simulink model "Stop_and_Wait"  (R2024b)
settings: Solver=FixedStepDiscrete  StartTime=0.0  StopTime=10.0  FixedStep=0.1  RelTol=1e-3  EnableMultiTasking=on
model workspace (MAT data in the model file):
  TxTree : serdes.internal.ibisami.ami.SerDesTree (value not decoded)
  input = Simulink.Bus
  input.Alignment = -1
  input.PreserveElementDimensions = 0
  input.Elements_internal = Simulink.BusElement
  input.Elements_internal.DimensionsMode = 'Fixed'
  input.Elements_internal.SamplingMode = 'Sample based'
  input.Elements_internal.SampleTime = -1
  input.Elements_internal.Name = 'in_data'
  input.Elements_internal.DataType_internal = 'uint8'
  input.Elements_internal.Complexity = 'real'
  input.Elements_internal.Dimensions = 1
  input.DataScope = 'Auto'
  output = Simulink.Bus
  output.Alignment = -1
  output.PreserveElementDimensions = 0
  output.Elements_internal = Simulink.BusElement
  output.Elements_internal.DimensionsMode = 'Fixed'
  output.Elements_internal.SamplingMode = 'Sample based'
  output.Elements_internal.SampleTime = -1
  output.Elements_internal.Name = 'out_data'
  output.Elements_internal.DataType_internal = 'uint8'
  output.Elements_internal.Complexity = 'real'
  output.Elements_internal.Dimensions = 1
  output.DataScope = 'Auto'
libraries: instrumentlib x4, dspbuff3 x1, simulink x1
settings Model: Creator=Amin  LastModifiedBy=Amin
settings SolverCC: PositivePriorityOrder=on
settings OptimizationCC: DefaultParameterBehavior=Inlined  EnhancedBackFolding=on  PassReuseOutputArgsAs=Individual arguments  ZeroExternalMemoryAtStartup=off  ZeroInternalMemoryAtStartup=off  MaxStackSize=64  OptimizeBlockOrder=speed  DifferentSizesBufferReuse=on  OptimizationCustomize=off  EfficientTunableParamExpr=on
settings DebuggingCC: ParameterTunabilityLossMsg=error
settings HardwareCC: ProdLongLongMode=on
settings ModelReferenceCC: ModelReferenceNumInstancesAllowed=Single
settings SFSimCC: LegacyBehaviorForPersistentVarInContinuousTime=on
settings RTWCC: Description=Embedded Coder  SystemTargetFile=ert.tlc  GenCodeOnly=on  PackageGeneratedCodeAndArtifacts=on  TemplateMakefile=ert_default_tmf  TargetLang=C++
settings CodeAppCC: ForceParamTrailComments=on  IgnoreCustomStorageClasses=off  OperatorAnnotations=on  SimulinkDataObjDesc=on  SFDataObjDesc=on  InsertBlockDesc=on
settings ERTTargetCC: CodeInterfacePackaging=C++ class  RootIOFormat=Structure reference  RTWCAPIRootIO=on  ERTCustomFileTemplate=example_file_process.tlc

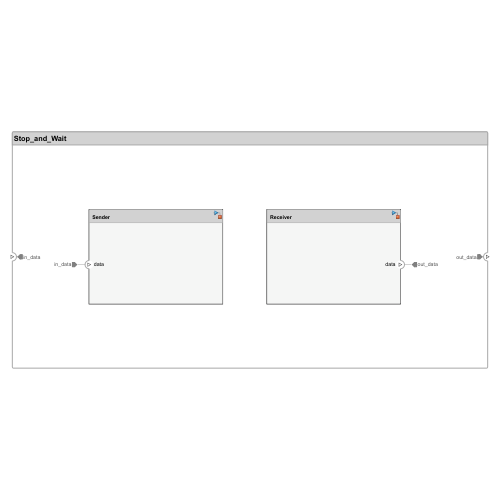
[thumbnail: Simulink's stored preview of the top-level diagram]
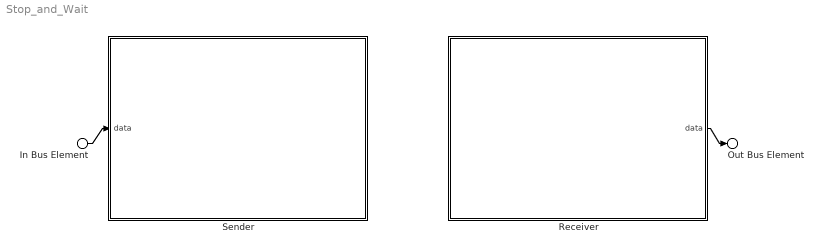
== system Stop_and_Wait ==
  In Bus Element : Inport  PortName=in_data
  Receiver : Subsystem
      settings: PortSchema="{\"entries\":[{\"content\":{\"headerSize\":26,\"margin\":15,\"minimumSpacing\":25,\"sides\":[{\"content\":{},\"type\":\"ConnectorPlacement.EquallySpacedRectSide\",\"uuid\":\"0072a2cb-bb3d-48a2-9d64-8e46ce8a1590\"},{\"content\":{\"connectorIds\":[\"Out1\"],\"side\":\"RIGHT\"},\"type\":\"ConnectorPlacement.EquallySpacedRectSide\",\"uuid\":\"e1929af3-b524-4cb4-8bf7-a19049f030de\"},{\"content\":{\"side\":\"TOP\"},\"type\":\"ConnectorPlacement.EquallySpacedRectSide\",\"uuid\":\"578aca91-09af-4b8b-8516-407c0ce534ed\"}]},\"type\":\"ConnectorPlacement.EquallySpacedConnector\",\"uuid\":\"ac7dd36b-d2bb-4d4d-8d57-dee4a1353f16\"}],\"packageUris\":[\"http://schema.mathworks.com/mf0/Connector/R2020b\"],\"version\":\"1.0\"}"
  Sender : Subsystem
      settings: PortSchema="{\"entries\":[{\"content\":{\"headerSize\":26,\"margin\":15,\"minimumSpacing\":25,\"sides\":[{\"content\":{\"connectorIds\":[\"In1\"]},\"type\":\"ConnectorPlacement.EquallySpacedRectSide\",\"uuid\":\"0072a2cb-bb3d-48a2-9d64-8e46ce8a1590\"},{\"content\":{\"side\":\"RIGHT\"},\"type\":\"ConnectorPlacement.EquallySpacedRectSide\",\"uuid\":\"e1929af3-b524-4cb4-8bf7-a19049f030de\"},{\"content\":{\"side\":\"TOP\"},\"type\":\"ConnectorPlacement.EquallySpacedRectSide\",\"uuid\":\"578aca91-09af-4b8b-8516-407c0ce534ed\"}]},\"type\":\"ConnectorPlacement.EquallySpacedConnector\",\"uuid\":\"ac7dd36b-d2bb-4d4d-8d57-dee4a1353f16\"}],\"packageUris\":[\"http://schema.mathworks.com/mf0/Connector/R2020b\"],\"version\":\"1.0\"}"
  Out Bus Element : Outport  PortName=out_data
  wires:
  In Bus Element/1 -> Sender/1(data)
  Receiver/1(data) -> Out Bus Element/1

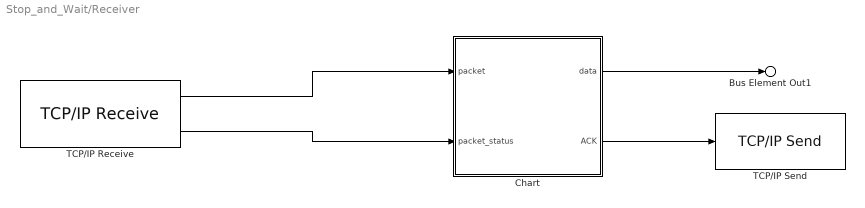
== system Stop_and_Wait/Receiver ==
  Chart : Stateflow chart  TreatAsAtomicUnit=on
  TCP/IP Receive : instrumentlib/TCP//IP Receive  Host=localhost  Port=54321  DataSize=[1, 1]  DataType=uint16  ASCIIFormatting=%f  Terminator=LF  CustomTerminator=10  ByteOrder=big-endian  EnableBlockingMode=off  Timeout=4  SampleTime=0.1  SimulateUsing=Interpreted execution
  TCP/IP Send : instrumentlib/TCP//IP Send  Host=localhost  Port=12345  ByteOrder=big-endian  EnableBlockingMode=off  Timeout=10  TransferDelay=off  SimulateUsing=Interpreted execution
  Bus Element Out1 : Outport  PortName=data  Element=out_data
  wires:
  Chart/2(ACK) -> TCP/IP Send/1
  Chart/1(data) -> Bus Element Out1/1
  TCP/IP Receive/1 -> Chart/1(packet)
  TCP/IP Receive/2 -> Chart/2(packet_status)

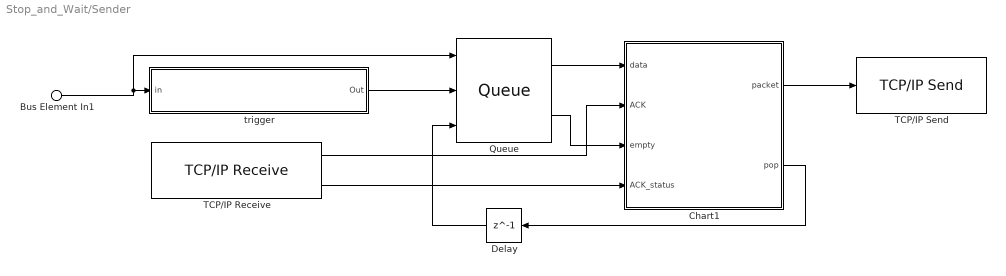
== system Stop_and_Wait/Sender ==
  Bus Element In1 : Inport  PortName=data  Element=in_data
  Chart1 : Stateflow chart  TreatAsAtomicUnit=on
  Delay : Delay  DelayLength=1
  Queue : dspbuff3/Queue  depth=256  trigger=Either edge  overflow=Warning  pes=Warning  eso=on  fso=off  nso=off  clr=off  clrOutport=off  adf=on
  TCP/IP Receive : instrumentlib/TCP//IP Receive  Host=localhost  Port=12345  DataSize=[1, 1]  DataType=uint8  ASCIIFormatting=%f  Terminator=LF  CustomTerminator=10  ByteOrder=big-endian  EnableBlockingMode=off  Timeout=4  SampleTime=0.1  SimulateUsing=Interpreted execution
  TCP/IP Send : instrumentlib/TCP//IP Send  Host=localhost  Port=54321  ByteOrder=big-endian  EnableBlockingMode=off  Timeout=4  TransferDelay=off  SimulateUsing=Interpreted execution
  trigger : Subsystem
  wires:
  TCP/IP Receive/1 -> Chart1/2(ACK)
  Chart1/1(packet) -> TCP/IP Send/1
  Queue/1 -> Chart1/1(data)
  Queue/2 -> Chart1/3(empty)
  Delay/1 -> Queue/3
  Chart1/2(pop) -> Delay/1
  trigger/1(Out) -> Queue/2
  TCP/IP Receive/2 -> Chart1/4(ACK_status)
  Bus Element In1/1 -> Queue/1, trigger/1(in)

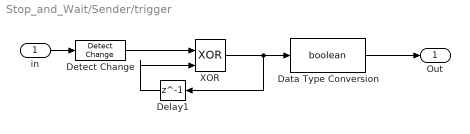
== system Stop_and_Wait/Sender/trigger ==
  in : Inport
  Data Type Conversion : DataTypeConversion  OutDataTypeStr=boolean  SaturateOnIntegerOverflow=off  RndMeth=Floor
  Delay1 : Delay  DelayLength=1
  Detect Change : simulink/Logic and Bit Operations/Detect Change  vinit=0  OutDataTypeStr=uint8
  XOR : Logic  Operator=XOR  IconShape=distinctive  AllPortsSameDT=off  OutDataTypeStr=boolean
  Out : Outport
  wires:
  XOR/1 -> Delay1/1, Data Type Conversion/1
  Delay1/1 -> XOR/2
  Detect Change/1 -> XOR/1
  Data Type Conversion/1 -> Out/1
  in/1 -> Detect Change/1

== stateflow chart Stop_and_Wait/Sender/Chart1 ==
  settings: stateMachineType=MEALY_MACHINE  executeAtInitialization=1
  state Dequeue
  state Send_packet
  state Wait_for_ack
  (default) -> Send_packet
  Dequeue -> Wait_for_ack : {packet = uint16(calculation(data, tag))}
  Send_packet -> Dequeue : [~empty]{send(pop)}
  Wait_for_ack -> Send_packet [order 2] : [ACK_status == 1 && checkACK(ACK, c_ACK)]{c_ACK = c_ACK + 1; tag = 1-tag;}
  Wait_for_ack -> Wait_for_ack [order 1] : [after(TIMEOUT, sec)]{packet = uint16(calculation(data, tag));}
  data: f function_output; ack function_input; check function_input; value function_input; t function_input; header function_output; polynomial function_input; input function_input uint8; output function_output uint16; c_tag function_input; value function_input; header function_output; polynomial function_input; TIMEOUT constant double =4; packet output uint16; data input uint8; ACK input uint8; c_ACK local uint8 =1; empty input boolean; ACK_status input; tag local single =1
  events: pop output EITHER_EDGE_EVENT
  function f = checkACK(ack, check):
    | function f = checkACK(ack, check)
    | 
    |     header = uint8(bitshift(ack, -4));
    |     ack_value = uint8(bitand(ack, 0x0F));
    |     if ack_crc(ack_value, 19) == header && ack_value == check
    |         f = true;
    |     else
    |         f = false;
    |     end
    |     
    | end
  function header = crc4(value, t, polynomial):
    | function header = crc4(value, t, polynomial)
    |         
    |     % Initialize the CRC register to 0
    |     crc = uint16(0);
    |     input = bitor(uint16(value), bitshift(uint16(t), 8));
    |         
    |     % Loop over each bit in the input byte (MSB first)
    |     for i = 8:-1:-4
    |         % XOR the MSB of the input with the MSB of the CRC register
    |         crc = bitxor(crc, bitand(bitshift(input, -i), 1));  % Shift input and XOR
    |             
    |         % If the MSB of the CRC is 1, perform the polynomial division (XOR)
    |         if bitget(crc, 5)  % Check if MSB (bit 5) of 8-bit crc is set
    |            crc = bitxor(crc, polynomial);  % Perform division by XOR with polynomial
    |         end
    |             
    |         if i ~= -4
    |             % Shift CRC register left by 1 bit
    |             crc = bitshift(crc, 1);
    |         end
    |     end
    |         
    |     
    |     % Final CRC value is the remainder in the lowest 4 bits
    |     header = uint8(bitand(crc, 15));  % Mask to get the lower 4 bits as the CRC result
    | end
  function output = calculation(input, c_tag):
    | function output = calculation(input, c_tag)
    |     
    |     
    |     output = bitor(bitor(uint16(input), bitshift(uint16(c_tag), 8)), bitshift(uint16(crc4(input, c_tag, 19)), 9));
    | 
    | end
  function header = ack_crc(value, polynomial):
    | function header = ack_crc(value, polynomial)
    |         
    |     % Initialize the CRC register to 0
    |     crc = uint8(0);
    |         
    |     % Loop over each bit in the input byte (MSB first)
    |     for i = 7:-1:-4
    |         % XOR the MSB of the input with the MSB of the CRC register
    |         crc = bitxor(crc, bitand(bitshift(value, -i), 1));  % Shift input and XOR
    |             
    |         % If the MSB of the CRC is 1, perform the polynomial division (XOR)
    |         if bitget(crc, 5)  % Check if MSB (bit 5) of 8-bit crc is set
    |            crc = bitxor(crc, polynomial);  % Perform division by XOR with polynomial
    |         end
    |             
    |         if i ~= -4
    |             % Shift CRC register left by 1 bit
    |             crc = bitshift(crc, 1);
    |         end
    |     end
    |         
    |     
    |     % Final CRC value is the remainder in the lowest 4 bits
    |     header = bitand(crc, 15);  % Mask to get the lower 4 bits as the CRC result
    | end

== stateflow chart Stop_and_Wait/Receiver/Chart ==
  settings: executeAtInitialization=1
  state state
  (default) -> state
  state -> state : [packet_status == 1 && check_packet(packet, tag)]{[data, ACK, c_ack] = send_data_ack(packet, c_ack); tag = 1-tag}
  data: f function_output; p function_input; t function_input; value function_input; crc_tag function_input; header function_output; polynomial function_input; p function_input; d function_output; a function_output; c function_input; nc function_output; value function_input; header function_output; polynomial function_input; data output uint8 =0; packet input uint16; ACK output uint8 =0; c_ack local uint8 =0; packet_status input boolean; tag local single =1
  function f = check_packet(p, t):
    | function f = check_packet(p, t)
    | 
    |     header = uint8(bitshift(p, -9));
    |     raw_data = uint8(bitand(p, 0x00FF));
    |     checktag = bitget(p, 9);
    |     if crc4(raw_data, tag, 19) == header && checktag == t
    |         f = true;
    |     else
    |         f = false;
    |     end
    |     
    | end
  function header = crc4(value, crc_tag, polynomial):
    | function header = crc4(value, crc_tag, polynomial)
    |         
    |     % Initialize the CRC register to 0
    |     crc = uint16(0);
    |     input = bitor(uint16(value), bitshift(uint16(crc_tag), 8));
    |         
    |     % Loop over each bit in the input byte (MSB first)
    |     for i = 8:-1:-4
    |         % XOR the MSB of the input with the MSB of the CRC register
    |         crc = bitxor(crc, bitand(bitshift(input, -i), 1));  % Shift input and XOR
    |             
    |         % If the MSB of the CRC is 1, perform the polynomial division (XOR)
    |         if bitget(crc, 5)  % Check if MSB (bit 5) of 8-bit crc is set
    |            crc = bitxor(crc, polynomial);  % Perform division by XOR with polynomial
    |         end
    |             
    |         if i ~= -4
    |             % Shift CRC register left by 1 bit
    |             crc = bitshift(crc, 1);
    |         end
    |     end
    |         
    |     
    |     % Final CRC value is the remainder in the lowest 4 bits
    |     header = uint8(bitand(crc, 15));  % Mask to get the lower 4 bits as the CRC result
    | end
  function [d, a, nc]= send_data_ack(p, c):
    | function [d, a, nc]= send_data_ack(p, c)
    | 
    |     d = uint8(bitand(p, 0x0011));
    | 
    |     if c == 16
    |         nc = uint8(0);
    |     else
    |         nc = uint8(c+1);
    |     end
    | 
    |     a = bitor(uint8(c+1), bitshift(uint8(ack_crc(uint8(c+1), 19)), 4));
    | 
    | end
  function header = ack_crc(value, polynomial):
    | function header = ack_crc(value, polynomial)
    |         
    |     % Initialize the CRC register to 0
    |     crc = uint8(0);
    |         
    |     % Loop over each bit in the input byte (MSB first)
    |     for i = 7:-1:-4
    |         % XOR the MSB of the input with the MSB of the CRC register
    |         crc = bitxor(crc, bitand(bitshift(value, -i), 1));  % Shift input and XOR
    |             
    |         % If the MSB of the CRC is 1, perform the polynomial division (XOR)
    |         if bitget(crc, 5)  % Check if MSB (bit 5) of 8-bit crc is set
    |            crc = bitxor(crc, polynomial);  % Perform division by XOR with polynomial
    |         end
    |             
    |         if i ~= -4
    |             % Shift CRC register left by 1 bit
    |             crc = bitshift(crc, 1);
    |         end
    |     end
    |         
    |     
    |     % Final CRC value is the remainder in the lowest 4 bits
    |     header = bitand(crc, 15);  % Mask to get the lower 4 bits as the CRC result
    | end
